simulink model "drone_main_dynamixal"  (R2023b)
settings: Solver=FixedStepAuto  StartTime=0.0  StopTime=inf  FixedStep=0.001  RelTol=1e-3
model workspace: external: MATLAB File drone_DataFile.m (data not in the file)
values from neighbouring files (symbols this model uses):
  coefthrust = 5.7199 / (max_prop^2)    (= 5.7199e-06)    [parameters.m]    (also in parameters.mat)
  coeftorque = 0.4008 / (max_prop^2)    (= 4.008e-07)    [parameters.m]    (also in parameters.mat)
  controlmatrix = pinv(controlmatrix)    [parameters.m]    (also in parameters.mat = [121408.493932 121408.493932 -121408.493932 -121408.493932 -)
  g = 9.8067    [parameters.m]    (also in parameters.mat)
  I = [0.0283    0.0003    0.0072 ... (first row only)    [parameters.m]    (also in parameters.mat = [0.0283  0.0003  0.0072; 0.0003  0.521  -0.0001; 0.0072  -0.)
  M =     [parameters.mat]
  m = pinv(mixmatrix)*b    [test.m]
  max_prop = 1000    [parameters.m]    (also in parameters.mat)
  poly_traj = pTraj    [trajectory.m]
  route = [0 0 1 0.5*pi ... (first row only)    [parameters.m]    (also in parameters.mat = [0 0 -3 -3 -3 3 0 3 3 4 4 4 ... (24 elements, 6x4)])
  smiData = struct    [drone_DataFile.m]
  total_mass = 2.1309    [parameters.m]    (also in parameters.mat)
undefined symbols (not defined in the file or in its folder): mass_total, X, Y, Z
libraries: sm_lib x173, slpidlib x90, nesl_utility x72, fl_lib x32, slctrl_autotuning x21, quadcopter_library x8, sdl_lib x8, simulink x3
(part 19 of 19)

== system drone_main_dynamixal/Controller2/positioncontroller/position_controller/move_pitch ==
  velocity : Inport
  position : Inport  Port=2
  setposition : Inport  Port=3
  transform : Inport  Port=4
  Closed-Loop PID Autotuner2 : slctrl_autotuning/Closed-Loop PID Autotuner  Commented=on  PIDType=PI  PIDForm=Parallel  TimeDomain=discrete-time  DiscreteTs=0.1  TuningTs=0.2  UseTuningTs=off  IntegratorFormula=Forward Euler  FilterFormula=Forward Euler  ContinuousTs=0.02  Bandwidth=1  UseExternalWC=off  TargetPM=60  UseExternalPM=off  UseExternalAchievedPM=off  ExperimentMode=Superposition  PlantType=Stable  PlantSign=Positive  AmpSine=1  UseExternalAmpSine=off  UseExternalFRD=off  UseExternalU0=off  UseCompanion=off  NotDeployTuningModule=off  UsePLCCoder=off  OutputMode=control action + perturbation  BlockDataType=double  UseConnectedPID=on  blockpath=[]  tunedP=0  tunedI=0  tunedD=0  tunedN=100  tunedPM=0  EstimationWindowSize=3  UseExternalTuningParams=off  SingleMultiRateVariant=SingleSamplingRate  NumEstimationPeriods=4  NumSettlingPeriods=2  NumOfPRBSPeriod=1  PRBSSignalOrder=12  ExperimentModeVariant=VariantSuperimposed  OutputChoice=VariantCandD
      settings: LibrarySourceBlock=slctrlblks/Autotuning/Closed-Loop PID Autotuner
  Closed-Loop PID Autotuner3 : slctrl_autotuning/Closed-Loop PID Autotuner  Commented=on  PIDType=PI  PIDForm=Parallel  TimeDomain=discrete-time  DiscreteTs=0.1  TuningTs=0.2  UseTuningTs=off  IntegratorFormula=Forward Euler  FilterFormula=Forward Euler  ContinuousTs=0.02  Bandwidth=1  UseExternalWC=off  TargetPM=60  UseExternalPM=off  UseExternalAchievedPM=off  ExperimentMode=Superposition  PlantType=Stable  PlantSign=Positive  AmpSine=1  UseExternalAmpSine=off  UseExternalFRD=off  UseExternalU0=off  UseCompanion=off  NotDeployTuningModule=off  UsePLCCoder=off  OutputMode=control action + perturbation  BlockDataType=double  UseConnectedPID=on  blockpath=[]  tunedP=0  tunedI=0  tunedD=0  tunedN=100  tunedPM=0  EstimationWindowSize=3  UseExternalTuningParams=off  SingleMultiRateVariant=SingleSamplingRate  NumEstimationPeriods=4  NumSettlingPeriods=2  NumOfPRBSPeriod=1  PRBSSignalOrder=12  ExperimentModeVariant=VariantSuperimposed  OutputChoice=VariantCandD
      settings: LibrarySourceBlock=slctrlblks/Autotuning/Closed-Loop PID Autotuner
  Constant : Constant  Value=0
  Demux : Demux  Outputs=2
  Demux1 : Demux  Outputs=2
  Demux2 : Demux  Outputs=3
  MATLAB Function : MATLAB Function  TreatAsAtomicUnit=on
  PID Controller1 : slpidlib/PID Controller  Controller=P  Form=Parallel  TimeDomain=Continuous-time  UseExternalTs=off  SampleTime=-1  IntegratorMethod=Forward Euler  FilterMethod=Forward Euler  ControllerParametersSource=internal  P=1  I=0.0001  UseKiTs=off  D=0.12  N=100  UseFilter=on  TunerSelectOption=Transfer Function Based (PID Tuner App)  InitialConditionSource=internal  InitialConditionForIntegrator=0  InitialConditionForFilter=0  DifferentiatorICPrevScaledInput=0  ExternalReset=none  TrackingMode=off  Kt=1  LimitOutput=off  SatLimitsSource=internal  UpperSaturationLimit=inf  LowerSaturationLimit=-inf  LinearizeAsGain=on  AntiWindupMode=none  Kb=1  LimitIntegrator=off  UpperIntegratorSaturationLimit=inf  LowerIntegratorSaturationLimit=-inf  POutMin=[]  POutMax=[]  IOutMin=[]  IOutMax=[]  DOutMin=[]  DOutMax=[]  NOutMin=[]  NOutMax=[]  SumOutMin=[]  SumOutMax=[]  SaturationOutMin=[]  SaturationOutMax=[]  PParamMin=[]  PParamMax=[]  IParamMin=[]  IParamMax=[]  DParamMin=[]  DParamMax=[]  NParamMin=[]  NParamMax=[]  KbParamMin=[]  KbParamMax=[]  KtParamMin=[]  KtParamMax=[]  KbOutMin=[]  KbOutMax=[]  KtOutMin=[]  KtOutMax=[]  IntegratorOutMin=[]  IntegratorOutMax=[]  FilterOutMin=[]  FilterOutMax=[]  SumI1OutMin=[]  SumI1OutMax=[]  SumI2OutMin=[]  SumI2OutMax=[]  SumI3OutMin=[]  SumI3OutMax=[]  SumI4OutMin=[]  SumI4OutMax=[]  SumDOutMin=[]  SumDOutMax=[]  DifferentiatorOutMin=[]  DifferentiatorOutMax=[]  FilterDiffOutCoefMin=[]  FilterDiffOutCoefMax=[]  ReciprocalOutMin=[]  ReciprocalOutMax=[]  SumDenOutMin=[]  SumDenOutMax=[]  SumNumOutMin=[]  SumNumOutMax=[]  DivideOutMin=[]  DivideOutMax=[]  UdiffTsProdOutMin=[]  UdiffTsProdOutMax=[]  NTsProdOutMin=[]  NTsProdOutMax=[]  UintegralTsProdOutMin=[]  UintegralTsProdOutMax=[]  UngainTsProdOutMin=[]  UngainTsProdOutMax=[]  ClampingZeroOutDataTypeStr=Inherit: Inherit via back propagation  ClampingZeroOutMin=[]  ClampingZeroOutMax=[]  FilterDenConstantOutDataTypeStr=Inherit: Inherit via back propagation  FilterDenConstantOutMin=[]  FilterDenConstantOutMax=[]  PCopyOutDataTypeStr=Inherit: Inherit via back propagation  PCopyOutMin=[]  PCopyOutMax=[]  NCopyOutDataTypeStr=Inherit: Inherit via back propagation  NCopyOutMin=[]  NCopyOutMax=[]  IntegratorContinuousStateAttributes=''  IntegratorStateMustResolveToSignalObject=off  IntegratorRTWStateStorageClass=Auto  FilterContinuousStateAttributes=''  FilterStateMustResolveToSignalObject=off  FilterRTWStateStorageClass=Auto  ParallelPVariant=InternalParameters  IdealPVariant=Disabled  IVariant=Disabled  DVariant=Disabled  IntegratorVariant=Disabled  SatVariant=Disabled  AWVariant=Disabled  PCopyVariant=Disabled  TRVariant=Disabled  FdbkBlocksVariant=Forward  IdealPFdbkVariant=Disabled  SatFdbkVariant=Disabled  DerivativeFilterVariant=Disabled  NVariant=Disabled  NCopyVariant=Disabled_SignalSpec  FilterICVariant=Disabled  IntegratorICVariant=Disabled  ExternalResetVariant=Disabled  TRSumVariant=Passthrough  SumFdbkVariant=Disabled  SumVariant=Passthrough_P  TsampFilterVariant=InternalTs  TsampNgainVariant=Passthrough  TsampIntegralVariant=Disabled_SignalSpec  ExternalSaturationOutDataTypeStr=Inherit: Same as second input
  PID Controller2 : slpidlib/PID Controller  Controller=P  Form=Parallel  TimeDomain=Continuous-time  UseExternalTs=off  SampleTime=-1  IntegratorMethod=Forward Euler  FilterMethod=Forward Euler  ControllerParametersSource=internal  P=1  I=0  UseKiTs=off  D=0  N=100  UseFilter=on  TunerSelectOption=Transfer Function Based (PID Tuner App)  InitialConditionSource=internal  InitialConditionForIntegrator=0  InitialConditionForFilter=0  DifferentiatorICPrevScaledInput=0  ExternalReset=none  TrackingMode=off  Kt=1  LimitOutput=off  SatLimitsSource=internal  UpperSaturationLimit=inf  LowerSaturationLimit=-inf  LinearizeAsGain=on  AntiWindupMode=none  Kb=1  LimitIntegrator=off  UpperIntegratorSaturationLimit=inf  LowerIntegratorSaturationLimit=-inf  POutMin=[]  POutMax=[]  IOutMin=[]  IOutMax=[]  DOutMin=[]  DOutMax=[]  NOutMin=[]  NOutMax=[]  SumOutMin=[]  SumOutMax=[]  SaturationOutMin=[]  SaturationOutMax=[]  PParamMin=[]  PParamMax=[]  IParamMin=[]  IParamMax=[]  DParamMin=[]  DParamMax=[]  NParamMin=[]  NParamMax=[]  KbParamMin=[]  KbParamMax=[]  KtParamMin=[]  KtParamMax=[]  KbOutMin=[]  KbOutMax=[]  KtOutMin=[]  KtOutMax=[]  IntegratorOutMin=[]  IntegratorOutMax=[]  FilterOutMin=[]  FilterOutMax=[]  SumI1OutMin=[]  SumI1OutMax=[]  SumI2OutMin=[]  SumI2OutMax=[]  SumI3OutMin=[]  SumI3OutMax=[]  SumI4OutMin=[]  SumI4OutMax=[]  SumDOutMin=[]  SumDOutMax=[]  DifferentiatorOutMin=[]  DifferentiatorOutMax=[]  FilterDiffOutCoefMin=[]  FilterDiffOutCoefMax=[]  ReciprocalOutMin=[]  ReciprocalOutMax=[]  SumDenOutMin=[]  SumDenOutMax=[]  SumNumOutMin=[]  SumNumOutMax=[]  DivideOutMin=[]  DivideOutMax=[]  UdiffTsProdOutMin=[]  UdiffTsProdOutMax=[]  NTsProdOutMin=[]  NTsProdOutMax=[]  UintegralTsProdOutMin=[]  UintegralTsProdOutMax=[]  UngainTsProdOutMin=[]  UngainTsProdOutMax=[]  ClampingZeroOutDataTypeStr=Inherit: Inherit via back propagation  ClampingZeroOutMin=[]  ClampingZeroOutMax=[]  FilterDenConstantOutDataTypeStr=Inherit: Inherit via back propagation  FilterDenConstantOutMin=[]  FilterDenConstantOutMax=[]  PCopyOutDataTypeStr=Inherit: Inherit via back propagation  PCopyOutMin=[]  PCopyOutMax=[]  NCopyOutDataTypeStr=Inherit: Inherit via back propagation  NCopyOutMin=[]  NCopyOutMax=[]  IntegratorContinuousStateAttributes=''  IntegratorStateMustResolveToSignalObject=off  IntegratorRTWStateStorageClass=Auto  FilterContinuousStateAttributes=''  FilterStateMustResolveToSignalObject=off  FilterRTWStateStorageClass=Auto  ParallelPVariant=InternalParameters  IdealPVariant=Disabled  IVariant=Disabled  DVariant=Disabled  IntegratorVariant=Disabled  SatVariant=Disabled  AWVariant=Disabled  PCopyVariant=Disabled  TRVariant=Disabled  FdbkBlocksVariant=Forward  IdealPFdbkVariant=Disabled  SatFdbkVariant=Disabled  DerivativeFilterVariant=Disabled  NVariant=Disabled  NCopyVariant=Disabled_SignalSpec  FilterICVariant=Disabled  IntegratorICVariant=Disabled  ExternalResetVariant=Disabled  TRSumVariant=Passthrough  SumFdbkVariant=Disabled  SumVariant=Passthrough_P  TsampFilterVariant=InternalTs  TsampNgainVariant=Passthrough  TsampIntegralVariant=Disabled_SignalSpec  ExternalSaturationOutDataTypeStr=Inherit: Same as second input
  PID Controller3 : slpidlib/PID Controller  Controller=PID  Form=Parallel  TimeDomain=Continuous-time  UseExternalTs=off  SampleTime=-1  IntegratorMethod=Forward Euler  FilterMethod=Forward Euler  ControllerParametersSource=internal  P=4  I=0.01  UseKiTs=off  D=2  N=100  UseFilter=on  TunerSelectOption=Transfer Function Based (PID Tuner App)  InitialConditionSource=internal  InitialConditionForIntegrator=0  InitialConditionForFilter=0  DifferentiatorICPrevScaledInput=0  ExternalReset=none  TrackingMode=off  Kt=1  LimitOutput=off  SatLimitsSource=internal  UpperSaturationLimit=inf  LowerSaturationLimit=-inf  LinearizeAsGain=on  AntiWindupMode=none  Kb=1  LimitIntegrator=off  UpperIntegratorSaturationLimit=inf  LowerIntegratorSaturationLimit=-inf  POutMin=[]  POutMax=[]  IOutMin=[]  IOutMax=[]  DOutMin=[]  DOutMax=[]  NOutMin=[]  NOutMax=[]  SumOutMin=[]  SumOutMax=[]  SaturationOutMin=[]  SaturationOutMax=[]  PParamMin=[]  PParamMax=[]  IParamMin=[]  IParamMax=[]  DParamMin=[]  DParamMax=[]  NParamMin=[]  NParamMax=[]  KbParamMin=[]  KbParamMax=[]  KtParamMin=[]  KtParamMax=[]  KbOutMin=[]  KbOutMax=[]  KtOutMin=[]  KtOutMax=[]  IntegratorOutMin=[]  IntegratorOutMax=[]  FilterOutMin=[]  FilterOutMax=[]  SumI1OutMin=[]  SumI1OutMax=[]  SumI2OutMin=[]  SumI2OutMax=[]  SumI3OutMin=[]  SumI3OutMax=[]  SumI4OutMin=[]  SumI4OutMax=[]  SumDOutMin=[]  SumDOutMax=[]  DifferentiatorOutMin=[]  DifferentiatorOutMax=[]  FilterDiffOutCoefMin=[]  FilterDiffOutCoefMax=[]  ReciprocalOutMin=[]  ReciprocalOutMax=[]  SumDenOutMin=[]  SumDenOutMax=[]  SumNumOutMin=[]  SumNumOutMax=[]  DivideOutMin=[]  DivideOutMax=[]  UdiffTsProdOutMin=[]  UdiffTsProdOutMax=[]  NTsProdOutMin=[]  NTsProdOutMax=[]  UintegralTsProdOutMin=[]  UintegralTsProdOutMax=[]  UngainTsProdOutMin=[]  UngainTsProdOutMax=[]  ClampingZeroOutDataTypeStr=Inherit: Inherit via back propagation  ClampingZeroOutMin=[]  ClampingZeroOutMax=[]  FilterDenConstantOutDataTypeStr=Inherit: Inherit via back propagation  FilterDenConstantOutMin=[]  FilterDenConstantOutMax=[]  PCopyOutDataTypeStr=Inherit: Inherit via back propagation  PCopyOutMin=[]  PCopyOutMax=[]  NCopyOutDataTypeStr=Inherit: Inherit via back propagation  NCopyOutMin=[]  NCopyOutMax=[]  IntegratorContinuousStateAttributes=''  IntegratorStateMustResolveToSignalObject=off  IntegratorRTWStateStorageClass=Auto  FilterContinuousStateAttributes=''  FilterStateMustResolveToSignalObject=off  FilterRTWStateStorageClass=Auto  ParallelPVariant=InternalParameters  IdealPVariant=Disabled  IVariant=InternalParameters  DVariant=InternalParameters  IntegratorVariant=Continuous  SatVariant=Disabled  AWVariant=Passthrough  PCopyVariant=Disabled  TRVariant=Disabled  FdbkBlocksVariant=Forward  IdealPFdbkVariant=Disabled  SatFdbkVariant=Disabled  DerivativeFilterVariant=ContFilter  NVariant=InternalParameters  NCopyVariant=Disabled  FilterICVariant=InternalICsFilter  IntegratorICVariant=InternalICs  ExternalResetVariant=Disabled  TRSumVariant=Passthrough  SumFdbkVariant=Disabled  SumVariant=Sum_PID  TsampFilterVariant=InternalTs  TsampNgainVariant=Passthrough  TsampIntegralVariant=Disabled_SignalSpec  ExternalSaturationOutDataTypeStr=Inherit: Same as second input
  PID Controller4 : slpidlib/PID Controller  Controller=PID  Form=Parallel  TimeDomain=Continuous-time  UseExternalTs=off  SampleTime=-1  IntegratorMethod=Forward Euler  FilterMethod=Forward Euler  ControllerParametersSource=internal  P=4  I=0.01  UseKiTs=off  D=2  N=100  UseFilter=on  TunerSelectOption=Transfer Function Based (PID Tuner App)  InitialConditionSource=internal  InitialConditionForIntegrator=0  InitialConditionForFilter=0  DifferentiatorICPrevScaledInput=0  ExternalReset=none  TrackingMode=off  Kt=1  LimitOutput=off  SatLimitsSource=internal  UpperSaturationLimit=inf  LowerSaturationLimit=-inf  LinearizeAsGain=on  AntiWindupMode=none  Kb=1  LimitIntegrator=off  UpperIntegratorSaturationLimit=inf  LowerIntegratorSaturationLimit=-inf  POutMin=[]  POutMax=[]  IOutMin=[]  IOutMax=[]  DOutMin=[]  DOutMax=[]  NOutMin=[]  NOutMax=[]  SumOutMin=[]  SumOutMax=[]  SaturationOutMin=[]  SaturationOutMax=[]  PParamMin=[]  PParamMax=[]  IParamMin=[]  IParamMax=[]  DParamMin=[]  DParamMax=[]  NParamMin=[]  NParamMax=[]  KbParamMin=[]  KbParamMax=[]  KtParamMin=[]  KtParamMax=[]  KbOutMin=[]  KbOutMax=[]  KtOutMin=[]  KtOutMax=[]  IntegratorOutMin=[]  IntegratorOutMax=[]  FilterOutMin=[]  FilterOutMax=[]  SumI1OutMin=[]  SumI1OutMax=[]  SumI2OutMin=[]  SumI2OutMax=[]  SumI3OutMin=[]  SumI3OutMax=[]  SumI4OutMin=[]  SumI4OutMax=[]  SumDOutMin=[]  SumDOutMax=[]  DifferentiatorOutMin=[]  DifferentiatorOutMax=[]  FilterDiffOutCoefMin=[]  FilterDiffOutCoefMax=[]  ReciprocalOutMin=[]  ReciprocalOutMax=[]  SumDenOutMin=[]  SumDenOutMax=[]  SumNumOutMin=[]  SumNumOutMax=[]  DivideOutMin=[]  DivideOutMax=[]  UdiffTsProdOutMin=[]  UdiffTsProdOutMax=[]  NTsProdOutMin=[]  NTsProdOutMax=[]  UintegralTsProdOutMin=[]  UintegralTsProdOutMax=[]  UngainTsProdOutMin=[]  UngainTsProdOutMax=[]  ClampingZeroOutDataTypeStr=Inherit: Inherit via back propagation  ClampingZeroOutMin=[]  ClampingZeroOutMax=[]  FilterDenConstantOutDataTypeStr=Inherit: Inherit via back propagation  FilterDenConstantOutMin=[]  FilterDenConstantOutMax=[]  PCopyOutDataTypeStr=Inherit: Inherit via back propagation  PCopyOutMin=[]  PCopyOutMax=[]  NCopyOutDataTypeStr=Inherit: Inherit via back propagation  NCopyOutMin=[]  NCopyOutMax=[]  IntegratorContinuousStateAttributes=''  IntegratorStateMustResolveToSignalObject=off  IntegratorRTWStateStorageClass=Auto  FilterContinuousStateAttributes=''  FilterStateMustResolveToSignalObject=off  FilterRTWStateStorageClass=Auto  ParallelPVariant=InternalParameters  IdealPVariant=Disabled  IVariant=InternalParameters  DVariant=InternalParameters  IntegratorVariant=Continuous  SatVariant=Disabled  AWVariant=Passthrough  PCopyVariant=Disabled  TRVariant=Disabled  FdbkBlocksVariant=Forward  IdealPFdbkVariant=Disabled  SatFdbkVariant=Disabled  DerivativeFilterVariant=ContFilter  NVariant=InternalParameters  NCopyVariant=Disabled  FilterICVariant=InternalICsFilter  IntegratorICVariant=InternalICs  ExternalResetVariant=Disabled  TRSumVariant=Passthrough  SumFdbkVariant=Disabled  SumVariant=Sum_PID  TsampFilterVariant=InternalTs  TsampNgainVariant=Passthrough  TsampIntegralVariant=Disabled_SignalSpec  ExternalSaturationOutDataTypeStr=Inherit: Same as second input
  PID Controller7 : slpidlib/PID Controller  Commented=on  Controller=PID  Form=Parallel  TimeDomain=Continuous-time  UseExternalTs=off  SampleTime=-1  IntegratorMethod=Forward Euler  FilterMethod=Forward Euler  ControllerParametersSource=internal  P=4  I=0.01  UseKiTs=off  D=2  N=100  UseFilter=on  TunerSelectOption=Transfer Function Based (PID Tuner App)  InitialConditionSource=internal  InitialConditionForIntegrator=0  InitialConditionForFilter=0  DifferentiatorICPrevScaledInput=0  ExternalReset=none  TrackingMode=off  Kt=1  LimitOutput=off  SatLimitsSource=internal  UpperSaturationLimit=inf  LowerSaturationLimit=-inf  LinearizeAsGain=on  AntiWindupMode=none  Kb=1  LimitIntegrator=off  UpperIntegratorSaturationLimit=inf  LowerIntegratorSaturationLimit=-inf  POutMin=[]  POutMax=[]  IOutMin=[]  IOutMax=[]  DOutMin=[]  DOutMax=[]  NOutMin=[]  NOutMax=[]  SumOutMin=[]  SumOutMax=[]  SaturationOutMin=[]  SaturationOutMax=[]  PParamMin=[]  PParamMax=[]  IParamMin=[]  IParamMax=[]  DParamMin=[]  DParamMax=[]  NParamMin=[]  NParamMax=[]  KbParamMin=[]  KbParamMax=[]  KtParamMin=[]  KtParamMax=[]  KbOutMin=[]  KbOutMax=[]  KtOutMin=[]  KtOutMax=[]  IntegratorOutMin=[]  IntegratorOutMax=[]  FilterOutMin=[]  FilterOutMax=[]  SumI1OutMin=[]  SumI1OutMax=[]  SumI2OutMin=[]  SumI2OutMax=[]  SumI3OutMin=[]  SumI3OutMax=[]  SumI4OutMin=[]  SumI4OutMax=[]  SumDOutMin=[]  SumDOutMax=[]  DifferentiatorOutMin=[]  DifferentiatorOutMax=[]  FilterDiffOutCoefMin=[]  FilterDiffOutCoefMax=[]  ReciprocalOutMin=[]  ReciprocalOutMax=[]  SumDenOutMin=[]  SumDenOutMax=[]  SumNumOutMin=[]  SumNumOutMax=[]  DivideOutMin=[]  DivideOutMax=[]  UdiffTsProdOutMin=[]  UdiffTsProdOutMax=[]  NTsProdOutMin=[]  NTsProdOutMax=[]  UintegralTsProdOutMin=[]  UintegralTsProdOutMax=[]  UngainTsProdOutMin=[]  UngainTsProdOutMax=[]  ClampingZeroOutDataTypeStr=Inherit: Inherit via back propagation  ClampingZeroOutMin=[]  ClampingZeroOutMax=[]  FilterDenConstantOutDataTypeStr=Inherit: Inherit via back propagation  FilterDenConstantOutMin=[]  FilterDenConstantOutMax=[]  PCopyOutDataTypeStr=Inherit: Inherit via back propagation  PCopyOutMin=[]  PCopyOutMax=[]  NCopyOutDataTypeStr=Inherit: Inherit via back propagation  NCopyOutMin=[]  NCopyOutMax=[]  IntegratorContinuousStateAttributes=''  IntegratorStateMustResolveToSignalObject=off  IntegratorRTWStateStorageClass=Auto  FilterContinuousStateAttributes=''  FilterStateMustResolveToSignalObject=off  FilterRTWStateStorageClass=Auto  ParallelPVariant=InternalParameters  IdealPVariant=Disabled  IVariant=InternalParameters  DVariant=InternalParameters  IntegratorVariant=Continuous  SatVariant=Disabled  AWVariant=Passthrough  PCopyVariant=Disabled  TRVariant=Disabled  FdbkBlocksVariant=Forward  IdealPFdbkVariant=Disabled  SatFdbkVariant=Disabled  DerivativeFilterVariant=ContFilter  NVariant=InternalParameters  NCopyVariant=Disabled  FilterICVariant=InternalICsFilter  IntegratorICVariant=InternalICs  ExternalResetVariant=Disabled  TRSumVariant=Passthrough  SumFdbkVariant=Disabled  SumVariant=Sum_PID  TsampFilterVariant=InternalTs  TsampNgainVariant=Passthrough  TsampIntegralVariant=Disabled_SignalSpec  ExternalSaturationOutDataTypeStr=Inherit: Same as second input
  Saturation : Saturate  UpperLimit=0.3  LowerLimit=-0.3
  Saturation1 : Saturate
  Scope{,1..4} (5 alike) : Scope
  Sum : Sum  Inputs=|-+
  Sum1 : Sum  Inputs=|-+
  Sum2 : Sum  Inputs=-+
  Sum3 : Sum  Inputs=-+
  Sum4 : Sum  Inputs=|++
  Sum5 : Sum  Inputs=|++
  To Workspace : ToWorkspace  VariableName=ex  SampleTime=-1
  To Workspace1 : ToWorkspace  VariableName=ey  SampleTime=-1
  roll : Outport
  pitch : Outport  Port=2
  yaw : Outport  Port=3
  vz : Outport  Port=4
  wires:
  Demux2/1 -> Closed-Loop PID Autotuner2/2, Sum2/1
  PID Controller4/1 -> Sum5/2, Closed-Loop PID Autotuner3/1
  Sum4/1 -> MATLAB Function/2(ex)
  MATLAB Function/2(pitch) -> Saturation1/1, Scope2/1
  Sum5/1 -> MATLAB Function/3(ey)
  transform/1 -> MATLAB Function/1(R)
  Sum3/1 -> PID Controller4/1
  Demux1/2 -> Sum1/2
  Constant/1 -> yaw/1
  Demux2/3 -> vz/1
  Sum1/1 -> PID Controller1/1, To Workspace1/1, Scope1/1
  PID Controller2/1 -> Sum2/2
  MATLAB Function/1(roll) -> Saturation/1
  Sum2/1 -> PID Controller3/1, Scope3/1
  Demux/2 -> Sum1/1
  position/1 -> Demux/1
  Demux2/2 -> Closed-Loop PID Autotuner3/2, Sum3/1
  Sum/1 -> PID Controller2/1, Scope4/1, Scope/1, To Workspace/1
  setposition/1 -> Demux1/1
  Demux1/1 -> Sum/2
  Closed-Loop PID Autotuner3/1 -> Sum5/1
  Demux/1 -> Sum/1
  PID Controller3/1 -> Closed-Loop PID Autotuner2/1, Sum4/2
  PID Controller1/1 -> Sum3/2
  velocity/1 -> Demux2/1
  Saturation/1 -> roll/1
  Closed-Loop PID Autotuner2/1 -> Sum4/1
  Saturation1/1 -> pitch/1

== system drone_main_dynamixal/plant/6 DOF/R to X-Y-Z Extrinsic/Unwrap ==
  angle : Inport
  w : Inport  Port=2
  Fcn1 : Fcn  Expr=u(2) + (2*(u(1) > u(2)) - 1)*2*pi*floor(abs(u(1)-u(2))/(2*pi) + 0.5)
  Gain1 : Gain  SaturateOnIntegerOverflow=on  OutDataTypeStr=Inherit: Same as input  ParamDataTypeStr=Inherit: Same as input
  Gain3 : Gain  SaturateOnIntegerOverflow=on  OutDataTypeStr=Inherit: Same as input  ParamDataTypeStr=Inherit: Same as input
  Gain4 : Gain  SaturateOnIntegerOverflow=on  OutDataTypeStr=Inherit: Same as input  ParamDataTypeStr=Inherit: Same as input
  Integrator : Integrator  InitialConditionSource=external  AbsoluteTolerance=1e-3  ZeroCross=off
  Mux : Mux  Inputs=2
  unwrapped : Outport
  wires:
  Gain1/1 -> Mux/2, Integrator/2
  Gain3/1 -> Integrator/1
  Fcn1/1 -> Gain4/1
  Mux/1 -> Fcn1/1
  Integrator/1 -> Mux/1
  angle/1 -> Gain1/1
  Gain4/1 -> unwrapped/1
  w/1 -> Gain3/1

== system drone_main_dynamixal/plant/6 DOF/Roll Pitch/Calculate aPitch ==
  Roll Angle : Inport
  uvec : Inport  Port=2
  Asin : Trigonometry  Operator=asin
  Cos : Trigonometry  Operator=cos
  Divide : Product  Inputs=*/
  Divide1 : Product  Inputs=*/
  Selector : Selector  InputPortWidth=3  IndexOptions=Index vector (dialog)  Indices=[3]  OutputSizes=1
  magnitude : Fcn  Expr=sqrt(u(1)*u(1)+u(2)*u(2)+u(3)*u(3))
  Angle : Outport  VectorParamsAs1DForOutWhenUnconnected=off
  wires:
  Divide1/1 -> Asin/1
  uvec/1 -> magnitude/1, Selector/1
  magnitude/1 -> Divide1/2
  Selector/1 -> Divide/1
  Roll Angle/1 -> Cos/1
  Asin/1 -> Angle/1
  Divide/1 -> Divide1/1
  Cos/1 -> Divide/2

== system drone_main_dynamixal/plant/6 DOF/Roll Pitch/Calculate aRoll ==
  uvec : Inport
  Demux : Demux  Outputs=3
  Mux : Mux  Inputs=2
  Trigonometric Function1 : Trigonometry  Operator=atan2
  magnitude : Fcn  Expr=sqrt(u(1)*u(1)+u(2)*u(2))
  Angle : Outport  VectorParamsAs1DForOutWhenUnconnected=off
  wires:
  Demux/2 -> Mux/2
  magnitude/1 -> Trigonometric Function1/2
  Mux/1 -> magnitude/1
  Demux/3 -> Trigonometric Function1/1
  Trigonometric Function1/1 -> Angle/1
  uvec/1 -> Demux/1
  Demux/1 -> Mux/1

== matlab function drone_main_dynamixal/plant/6 DOF/MATLAB Function ==
  data: u input; y output
function y = fcn(u)
y = quat2rotm(u');
end

== matlab function drone_main_dynamixal/Controller/positioncontroller/MATLAB Function ==
  data: u input; y output
function y = fcn(u)
y = rotm2eul(u, 'XYZ');
end

== matlab function drone_main_dynamixal/Controller/MATLAB Function ==
  data: u input; theta input; M input; p output
function p = fcn(u, theta, M)
Lx = M.Lx;
Ly = M.Ly;
Lz = M.Lz;
coefthrust = M.coefthrust;
coeftorque = M.coeftorque;
platformmass = M.platformmass;
total_mass = M.total_mass;
total_cg = M.total_cg;
Lyf = Ly;
Lyb = Ly;

c = cos(theta);
s = sin(theta);
% PMatrix = [-Ly*coefthrust, -Ly*coefthrust, -Ly*coefthrust, -Ly*coefthrust, Ly*coefthrust, -Lz*coefthrust, Ly*coefthrust, -Lz*coefthrust, Ly*coefthrust, -Lz*coefthrust, Ly*coefthrust, -Lz*coefthrust;];
% pitch = u(2);
% thetaD = pinv(PMatrix) * pitch;
% thetaD = atan2(thetaD(end), thetaD(end-1));
% c = cos(thetaD);
% s = sin(thetaD);
% dcg = total_mass/platformmass*d+Ly+total_cg;
% Lyf = Lyf - dcg;
% Lyb = Lyb + dcg;

controlmatrix = [Lx*coefthrust, Lx*coefthrust, -Lx*coefthrust, -Lx*coefthrust, -Lx*coefthrust*c+coeftorque*s, -Lx*coefthrust*c-coeftorque*s, Lx*coefthrust*c-coeftorque*s, Lx*coefthrust*c+coeftorque*s,0;
                -Lyf*coefthrust, -Lyf*coefthrust, -Lyf*coefthrust, -Lyf*coefthrust, (Lyb*c-Lz*s)*coefthrust, (Lyb*c-Lz*s)*coefthrust, (Lyb*c-Lz*s)*coefthrust, (Lyb*c-Lz*s)*coefthrust,1;
                coeftorque, -coeftorque, -coeftorque, coeftorque, coeftorque*c, -coeftorque*c, -coeftorque*c, coeftorque*c,0;
                coefthrust,coefthrust,coefthrust,coefthrust,coefthrust*c,coefthrust*c,coefthrust*c,coefthrust*c,0];
controlmatrix = pinv(controlmatrix);
output = controlmatrix * u;
thrust = u(4);
d = output(end) / thrust;
Xplatform = platformmass/(total_mass)*(d-Ly-total_cg);
p = Xplatform;
end

== matlab function drone_main_dynamixal/Controller/positioncontroller/position_controller/move_pitch/MATLAB Function ==
  data: R input; roll output; ex input; ey input; pitch output
function [roll, pitch] = positioncontrol(R, ex, ey)
A = [0 -1 0 
     1 0 0];
E = [ex;ey;0];
out = A * R * E;
roll = out(1);
pitch = out(2);
end

== matlab function drone_main_dynamixal/Controller/MATLAB Function1 ==
  data: u input; y output
function y = fcn(u)
y = rotm2eul(u,'XYZ');
end

== matlab function drone_main_dynamixal/Controller/positioncontroller/position_controller/move_axis/MATLAB Function1 ==
  data: roll output; ex input; ey input; pitch output
function [roll, pitch] = positioncontrol(ex, ey)
A = [0 -1 0 
     1 0 0];
E = [ex;ey;0];
% R = inv(R);
% out = A * R * E;
% out = E' * R * A';
out = E' * A';
roll = out(1);
pitch = out(2);
end

== matlab function drone_main_dynamixal/Controller/positioncontroller/position_controller/move_axis/MATLAB Function2 ==
  data: R input; u input; y output
function y = fcn(R,u)
y = u'*R;
end

== matlab function drone_main_dynamixal/Controller/positioncontroller/position_controller/move_axis/MATLAB Function3 ==
  data: R input; u input; y output
function y = fcn(R,u)
y = u'*R;
end

== matlab function drone_main_dynamixal/Controller/positioncontroller/position_controller/move_axis/MATLAB Function4 ==
  data: R input; u input; y output
function y = fcn(R,u)
y = u'*R;
end

== matlab function drone_main_dynamixal/Controller1/MATLAB Function ==
  data: u input; theta input; d input; y output; M input
function y = fcn(u, theta, d, M)
Lx = M.Lx;
Ly = M.Ly;
Lz = M.Lz;
coefthrust = M.coefthrust;
coeftorque = M.coeftorque;
platformmass = M.platformmass;
total_mass = M.total_mass;
total_cg = M.total_cg;
Lyf = Ly;
Lyb = Ly;

c = cos(theta);
s = sin(theta);
% PMatrix = [-Ly*coefthrust, -Ly*coefthrust, -Ly*coefthrust, -Ly*coefthrust, Ly*coefthrust, -Lz*coefthrust, Ly*coefthrust, -Lz*coefthrust, Ly*coefthrust, -Lz*coefthrust, Ly*coefthrust, -Lz*coefthrust;];
% pitch = u(2);
% thetaD = pinv(PMatrix) * pitch;
% thetaD = atan2(thetaD(end), thetaD(end-1));
% c = cos(thetaD);
% s = sin(thetaD);
dcg = total_mass/platformmass*d+Ly+total_cg;
Lyf = Lyf - dcg;
Lyb = Lyb + dcg;
controlmatrix = [Lx*coefthrust, Lx*coefthrust, -Lx*coefthrust, -Lx*coefthrust, -Lx*coefthrust*c+coeftorque*s, -Lx*coefthrust*c-coeftorque*s, Lx*coefthrust*c-coeftorque*s, Lx*coefthrust*c+coeftorque*s;
                -Lyf*coefthrust, -Lyf*coefthrust, -Lyf*coefthrust, -Lyf*coefthrust, (Lyb*c-Lz*s)*coefthrust, (Lyb*c-Lz*s)*coefthrust, (Lyb*c-Lz*s)*coefthrust, (Lyb*c-Lz*s)*coefthrust;
                coeftorque, -coeftorque, -coeftorque, coeftorque, coeftorque*c, -coeftorque*c, -coeftorque*c, coeftorque*c;
                coefthrust,coefthrust,coefthrust,coefthrust,coefthrust*c,coefthrust*c,coefthrust*c,coefthrust*c];
controlmatrix = pinv(controlmatrix);
y = controlmatrix * u;
% d = output(end) / thrust;
% Xplatform = platformmass/(total_mass)*(d-Ly-total_cg);
% y = output(1:8);
% p = Xplatform;
end

== matlab function drone_main_dynamixal/Controller1/MATLAB Function1 ==
  data: u input; y output
function y = fcn(u)
y = rotm2eul(u,'XYZ');
end

== matlab function drone_main_dynamixal/Controller1/MATLAB Function2 ==
  data: u input; y output; M input
function y = fcn(u, M)
y = M * u;
end

== matlab function drone_main_dynamixal/Controller1/MATLAB Function3 ==
  data: d input; maxtheta output; M input
function maxtheta = fcn(d,M)
Ly = M.Ly;
Lz = M.Lz;
total_mass = M.total_mass;
platformmass = M.platformmass;
total_cg = M.total_cg;
dcg = total_mass/platformmass*d+Ly+total_cg;
maxtheta = atan2(Ly+dcg,Lz) - 0.2;
end

== matlab function drone_main_dynamixal/Controller1/attitudecontroller/MATLAB Function ==
  data: v input; y output; I input
function y = matrixmutiply(v, I)
y = I * v;
end

== matlab function drone_main_dynamixal/Controller1/positioncontroller/MATLAB Function ==
  data: u input; y output
function y = fcn(u)
y = rotm2eul(u, 'XYZ');
end

== matlab function drone_main_dynamixal/Controller1/positioncontroller/MATLAB Function1 ==
  data: u input; y output; m input; g input; e input
function y = fcn(u, m, g, e)
y = m * (g + e) / cos(u(1)) / cos(u(2));
end

== matlab function drone_main_dynamixal/Controller1/positioncontroller/position_controller/Subsystem1/MATLAB Function ==
  data: R input; roll output; ex input; ey input; pitch output
function [roll, pitch] = positioncontrol(R, ex, ey)
A = [0 -1 0 
     1 0 0];
E = [ex;ey;0];
out = A * R * E;
roll = out(1);
pitch = out(2);
end

== matlab function drone_main_dynamixal/Controller1/positioncontroller/position_controller/move_axis/MATLAB Function ==
  data: R input; roll output; ex input; ey input; pitch output
function [roll, pitch] = positioncontrol(R, ex, ey)
A = [0 -1 0 
     1 0 0];
E = [ex;ey;0];
% R = inv(R);
% out = A * R * E;
% out = E' * R * A';
out = E' * A';
roll = out(1);
pitch = out(2);
end

== matlab function drone_main_dynamixal/Controller1/positioncontroller/position_controller/move_axis/MATLAB Function1 ==
  data: R input; roll output; ex input; ey input; pitch output
function [roll, pitch] = positioncontrol(R, ex, ey)
A = [0 -1 0 
     1 0 0];
E = [ex;ey;0];
% R = inv(R);
% out = A * R * E;
% out = E' * R * A';
out = E' * A';
roll = out(1);
pitch = out(2);
end

== matlab function drone_main_dynamixal/Controller1/positioncontroller/position_controller/move_axis/MATLAB Function2 ==
  data: R input; u input; y output
function y = fcn(R,u)
y = u'*R;
end

== matlab function drone_main_dynamixal/Controller1/positioncontroller/position_controller/move_axis/MATLAB Function3 ==
  data: R input; u input; y output
function y = fcn(R,u)
y = u'*R;
end

== matlab function drone_main_dynamixal/Controller1/positioncontroller/position_controller/move_axis/MATLAB Function4 ==
  data: R input; u input; y output
function y = fcn(R,u)
y = u'*R;
end

== matlab function drone_main_dynamixal/Controller1/positioncontroller/position_controller/move_pitch/MATLAB Function ==
  data: R input; roll output; ex input; ey input; pitch output
function [roll, pitch] = positioncontrol(R, ex, ey)
A = [0 -1 0 
     1 0 0];
E = [ex;ey;0];
out = A * R * E;
roll = out(1);
pitch = out(2);
end

== matlab function drone_main_dynamixal/Controller2/Subsystem1/MATLAB Function1 ==
  data: roll input size=1; pitch input size=1; yaw input size=1; er output size=[3 1]; R input size=[3 3]
function er = lee(roll, pitch, yaw, R)

Rd = eul2rotm([yaw pitch roll], 'ZYX');

P = 1/2 * (Rd.' * R - R.' * Rd) ;

er = [P(3,2) ; P(1,3) ; P(2,1)] ;

== matlab function drone_main_dynamixal/Controller2/position controller/compute_roll_pitch ==
  data: F_d input; roll output; yaw_d input; pitch output
function [roll, pitch] = compute_roll_pitch(F_d, yaw_d)

yaw_dt = yaw_d + pi/2;
uyt = [cos(yaw_dt); sin(yaw_dt); 0];
uz = F_d/norm(F_d);
ux = cross(uyt, uz);
uy = cross(uz, ux);

attitude = rotm2eul([ux uy uz], 'ZYX');

roll = attitude(3);
pitch = attitude(2);

== matlab function drone_main_dynamixal/Controller2/MATLAB Function ==
  data: u input; theta input; d input; y output; M input
function y = fcn(u, theta, d, M)
Lx = M.Lx;
Ly = M.Ly;
Lz = M.Lz;
coefthrust = M.coefthrust;
coeftorque = M.coeftorque;
platformmass = M.platformmass;
total_mass = M.total_mass;
total_cg = M.total_cg;
Lyf = Ly;
Lyb = Ly;

c = cos(theta);
s = sin(theta);
% PMatrix = [-Ly*coefthrust, -Ly*coefthrust, -Ly*coefthrust, -Ly*coefthrust, Ly*coefthrust, -Lz*coefthrust, Ly*coefthrust, -Lz*coefthrust, Ly*coefthrust, -Lz*coefthrust, Ly*coefthrust, -Lz*coefthrust;];
% pitch = u(2);
% thetaD = pinv(PMatrix) * pitch;
% thetaD = atan2(thetaD(end), thetaD(end-1));
% c = cos(thetaD);
% s = sin(thetaD);
dcg = total_mass/platformmass*d+Ly+total_cg;
Lyf = Lyf - dcg;
Lyb = Lyb + dcg;
controlmatrix = [Lx*coefthrust, Lx*coefthrust, -Lx*coefthrust, -Lx*coefthrust, -Lx*coefthrust*c+coeftorque*s, -Lx*coefthrust*c-coeftorque*s, Lx*coefthrust*c-coeftorque*s, Lx*coefthrust*c+coeftorque*s;
                -Lyf*coefthrust, -Lyf*coefthrust, -Lyf*coefthrust, -Lyf*coefthrust, (Lyb*c-Lz*s)*coefthrust, (Lyb*c-Lz*s)*coefthrust, (Lyb*c-Lz*s)*coefthrust, (Lyb*c-Lz*s)*coefthrust;
                coeftorque, -coeftorque, -coeftorque, coeftorque, coeftorque*c, -coeftorque*c, -coeftorque*c, coeftorque*c;
                coefthrust,coefthrust,coefthrust,coefthrust,coefthrust*c,coefthrust*c,coefthrust*c,coefthrust*c];
controlmatrix = pinv(controlmatrix);
y = controlmatrix * u;
% d = output(end) / thrust;
% Xplatform = platformmass/(total_mass)*(d-Ly-total_cg);
% y = output(1:8);
% p = Xplatform;
end

== matlab function drone_main_dynamixal/Controller2/MATLAB Function1 ==
  data: u input; y output
function y = fcn(u)
y = rotm2eul(u,'XYZ');
end

== matlab function drone_main_dynamixal/Controller2/MATLAB Function2 ==
  data: u input; y output; M input
function y = fcn(u, M)
y = M * u;
end

== matlab function drone_main_dynamixal/Controller2/MATLAB Function3 ==
  data: d input; maxtheta output; M input
function maxtheta = fcn(d,M)
Ly = M.Ly;
Lz = M.Lz;
total_mass = M.total_mass;
platformmass = M.platformmass;
total_cg = M.total_cg;
dcg = total_mass/platformmass*d+Ly+total_cg;
maxtheta = atan2(Ly+dcg,Lz) - 0.2;
end

== matlab function drone_main_dynamixal/Controller2/attitudecontroller/MATLAB Function ==
  data: v input; y output; I input
function y = matrixmutiply(v, I)
y = I * v;
end

== matlab function drone_main_dynamixal/Controller2/positioncontroller/MATLAB Function ==
  data: u input; y output
function y = fcn(u)
y = rotm2eul(u, 'XYZ');
end

== matlab function drone_main_dynamixal/Controller2/positioncontroller/MATLAB Function1 ==
  data: u input; y output; m input; g input; e input
function y = fcn(u, m, g, e)
y = m * (g + e) / cos(u(1)) / cos(u(2));
end

== matlab function drone_main_dynamixal/Controller2/positioncontroller/position_controller/Subsystem1/MATLAB Function ==
  data: R input; roll output; ex input; ey input; pitch output
function [roll, pitch] = positioncontrol(R, ex, ey)
A = [0 -1 0 
     1 0 0];
E = [ex;ey;0];
out = A * R * E;
roll = out(1);
pitch = out(2);
end

== matlab function drone_main_dynamixal/Controller2/positioncontroller/position_controller/move_axis/MATLAB Function ==
  data: R input; roll output; ex input; ey input; pitch output
function [roll, pitch] = positioncontrol(R, ex, ey)
A = [0 -1 0 
     1 0 0];
E = [ex;ey;0];
% R = inv(R);
% out = A * R * E;
% out = E' * R * A';
out = E' * A';
roll = out(1);
pitch = out(2);
end

== matlab function drone_main_dynamixal/Controller2/positioncontroller/position_controller/move_axis/MATLAB Function1 ==
  data: R input; roll output; ex input; ey input; pitch output
function [roll, pitch] = positioncontrol(R, ex, ey)
A = [0 -1 0 
     1 0 0];
E = [ex;ey;0];
% R = inv(R);
% out = A * R * E;
% out = E' * R * A';
out = E' * A';
roll = out(1);
pitch = out(2);
end

== matlab function drone_main_dynamixal/Controller2/positioncontroller/position_controller/move_axis/MATLAB Function2 ==
  data: R input; u input; y output
function y = fcn(R,u)
y = u'*R;
end

== matlab function drone_main_dynamixal/Controller2/positioncontroller/position_controller/move_axis/MATLAB Function3 ==
  data: R input; u input; y output
function y = fcn(R,u)
y = u'*R;
end

== matlab function drone_main_dynamixal/Controller2/positioncontroller/position_controller/move_axis/MATLAB Function4 ==
  data: R input; u input; y output
function y = fcn(R,u)
y = u'*R;
end

== matlab function drone_main_dynamixal/Controller2/positioncontroller/position_controller/move_pitch/MATLAB Function ==
  data: R input; roll output; ex input; ey input; pitch output
function [roll, pitch] = positioncontrol(R, ex, ey)
A = [0 -1 0 
     1 0 0];
E = [ex;ey;0];
out = A * R * E;
roll = out(1);
pitch = out(2);
end

== matlab function drone_main_dynamixal/Controller2/Subsystem1/MATLAB Function ==
  data: v input; y output; I input
function y = matrixmutiply(v, I)
y = I * v;
end

== matlab function drone_main_dynamixal/Controller/MATLAB Function4 ==
  data: u input; theta input; d input; y output; M input
function y = fcn(u, theta, d, M)
Lx = M.Lx;
Ly = M.Ly;
Lz = M.Lz;
coefthrust = M.coefthrust;
coeftorque = M.coeftorque;
platformmass = M.platformmass;
total_mass = M.total_mass;
total_cg = M.total_cg;
Lyf = Ly;
Lyb = Ly;

c = cos(theta);
s = sin(theta);
% PMatrix = [-Ly*coefthrust, -Ly*coefthrust, -Ly*coefthrust, -Ly*coefthrust, Ly*coefthrust, -Lz*coefthrust, Ly*coefthrust, -Lz*coefthrust, Ly*coefthrust, -Lz*coefthrust, Ly*coefthrust, -Lz*coefthrust;];
% pitch = u(2);
% thetaD = pinv(PMatrix) * pitch;
% thetaD = atan2(thetaD(end), thetaD(end-1));
% c = cos(thetaD);
% s = sin(thetaD);
dcg = total_mass/platformmass*d+Ly+total_cg;
Lyf = Lyf - dcg;
Lyb = Lyb + dcg;

controlmatrix = [Lx*coefthrust, Lx*coefthrust, -Lx*coefthrust, -Lx*coefthrust, -Lx*coefthrust*c+coeftorque*s, -Lx*coefthrust*c-coeftorque*s, Lx*coefthrust*c-coeftorque*s, Lx*coefthrust*c+coeftorque*s;
                -Lyf*coefthrust, -Lyf*coefthrust, -Lyf*coefthrust, -Lyf*coefthrust, (Lyb*c-Lz*s)*coefthrust, (Lyb*c-Lz*s)*coefthrust, (Lyb*c-Lz*s)*coefthrust, (Lyb*c-Lz*s)*coefthrust;
                coeftorque, -coeftorque, -coeftorque, coeftorque, coeftorque*c, -coeftorque*c, -coeftorque*c, coeftorque*c;
                coefthrust,coefthrust,coefthrust,coefthrust,coefthrust*c,coefthrust*c,coefthrust*c,coefthrust*c];
controlmatrix = pinv(controlmatrix);
y = controlmatrix * u;
% d = output(end) / thrust;
% Xplatform = platformmass/(total_mass)*(d-Ly-total_cg);
% y = output(1:8);
% p = Xplatform;
end

== matlab function drone_main_dynamixal/Controller/MATLAB Function5 ==
  data: u input; theta input; d input; y output; M input; p output
function [y,p] = fcn(u, theta, d, M)
Lx = M.Lx;
Ly = M.Ly;
Lz = M.Lz;
coefthrust = M.coefthrust;
coeftorque = M.coeftorque;
platformmass = M.platformmass;
total_mass = M.total_mass;
total_cg = M.total_cg;
Lyf = Ly;
Lyb = Ly;

c = cos(theta);
s = sin(theta);

controlmatrix = [Lx*coefthrust, Lx*coefthrust, -Lx*coefthrust, -Lx*coefthrust, -Lx*coefthrust*c+coeftorque*s, -Lx*coefthrust*c-coeftorque*s, Lx*coefthrust*c-coeftorque*s, Lx*coefthrust*c+coeftorque*s,0;
                -Lyf*coefthrust, -Lyf*coefthrust, -Lyf*coefthrust, -Lyf*coefthrust, (Lyb*c-Lz*s)*coefthrust, (Lyb*c-Lz*s)*coefthrust, (Lyb*c-Lz*s)*coefthrust, (Lyb*c-Lz*s)*coefthrust,1;
                coeftorque, -coeftorque, -coeftorque, coeftorque, coeftorque*c, -coeftorque*c, -coeftorque*c, coeftorque*c,0;
                coefthrust,coefthrust,coefthrust,coefthrust,coefthrust*c,coefthrust*c,coefthrust*c,coefthrust*c,0];
controlmatrix = pinv(controlmatrix);
output = controlmatrix * u;
thrust = u(4);
p = output(end) / thrust;
Xplatform = total_mass/(platformmass)*(p-Ly-total_cg);
p = Xplatform;
if p>0.4
    p=0.4;
elseif p<-0.03
    p=-0.03;
end

dcg = platformmass/total_mass*d+Ly+total_cg;
Lyf = Lyf - dcg;
Lyb = Lyb + dcg;

controlmatrix = [Lx*coefthrust, Lx*coefthrust, -Lx*coefthrust, -Lx*coefthrust, -Lx*coefthrust*c+coeftorque*s, -Lx*coefthrust*c-coeftorque*s, Lx*coefthrust*c-coeftorque*s, Lx*coefthrust*c+coeftorque*s;
                -Lyf*coefthrust, -Lyf*coefthrust, -Lyf*coefthrust, -Lyf*coefthrust, (Lyb*c-Lz*s)*coefthrust, (Lyb*c-Lz*s)*coefthrust, (Lyb*c-Lz*s)*coefthrust, (Lyb*c-Lz*s)*coefthrust;
                coeftorque, -coeftorque, -coeftorque, coeftorque, coeftorque*c, -coeftorque*c, -coeftorque*c, coeftorque*c;
                coefthrust,coefthrust,coefthrust,coefthrust,coefthrust*c,coefthrust*c,coefthrust*c,coefthrust*c];
controlmatrix = pinv(controlmatrix);
y = controlmatrix * u;
end

== matlab function drone_main_dynamixal/MATLAB Function ==
  data: unext input; u input; y output
function y = fcn(unext, u)
y = atan2(unext(2)-u(2), unext(1)-u(1));
end

== stateflow chart drone_main_dynamixal/waypoint navigation (Ex. 6.1 and 7.1)1 ==
  state go
    pd = [r(i, 1) ; r(i, 2) ; r(i, 3)]
    yawd = r(i, 4)
  (default) -> go : {i = 1}
  go -> (junction 26) : [reached(pd, p, yawd, yaw)]
  (junction 26) -> go : [i < size(r, 1)]{i = i + 1}
  data: setpoint_position function_input; position function_input; is_reached function_output; yawd function_input; yaw function_input; yawd output; r input; yaw input; i local; p input; pd output size=[3 1]
  function is_reached = reached(setpoint_position, position, yawd, yaw):
    | function is_reached = reached(setpoint_position, position, yawd, yaw)
    | is_reached = (norm(position - setpoint_position) < 0.05) && (norm(yawd - yaw) < 0.05);

== matlab function drone_main_dynamixal/Controller/positioncontroller/position_controller/move_axis/MATLAB Function5 ==
  data: R input; u input; y output
function y = fcn(R,u)
y = u'*R;
end

== matlab function drone_main_dynamixal/Controller/positioncontroller/position_controller/move_axis/MATLAB Function6 ==
  data: R input; u input; y output
function y = fcn(R,u)
y = u'*R;
end

== matlab function drone_main_dynamixal/Controller/positioncontroller/MATLAB Function1 ==
  data: u input; y output; m input; g input; e input
function y = fcn(u, m, g, e)
y = m * (g + e) / cos(u(1)) / cos(u(2));
end

== matlab function drone_main_dynamixal/Controller/attitudecontroller/MATLAB Function ==
  data: v input; y output; I input
function y = matrixmutiply(v, I)
y = I * v;
end

== matlab function drone_main_dynamixal/Controller/MATLAB Function2 ==
  data: u input; y output; M input
function y = fcn(u, M)
y = M * u;
end

== matlab function drone_main_dynamixal/Controller/positioncontroller/position_controller/move_axis/MATLAB Function ==
  data: roll output; ex input; ey input; pitch output
function [roll, pitch] = positioncontrol(ex, ey)
A = [0 -1 0 
     1 0 0];
E = [ex;ey;0];
% R = inv(R);
% out = A * R * E;
% out = E' * R * A';
out = E' * A';
roll = out(1);
pitch = out(2);
end

== matlab function drone_main_dynamixal/Controller/positioncontroller/position_controller/Subsystem1/MATLAB Function ==
  data: R input; roll output; ex input; ey input; pitch output
function [roll, pitch] = positioncontrol(R, ex, ey)
A = [0 -1 0 
     1 0 0];
E = [ex;ey;0];
out = A * R * E;
roll = out(1);
pitch = out(2);
end
